simulink model "geuus"  (R2017b)
settings: Solver=VariableStepAuto  StartTime=0.0  StopTime=10.0  RelTol=1e-3
values from neighbouring files (symbols this model uses):
  d2hhh1 = fnval(fnder(fnder(sp1)),vvv1)    [feedbackcontrolcal.m]
  d2hhh2 = fnval(fnder(fnder(sp2)),vvv2)    [feedbackcontrolcal.m]
  dhhh1 = fnval(fnder(sp1),vvv1)    [feedbackcontrolcal.m]
  dhhh2 = fnval(fnder(sp2),vvv2)    [feedbackcontrolcal.m]
  hhh1 = altitude(1:19)*1000    [feedbackcontrolcal.m]
  hhh2 = altitude(19:end)*1000    [feedbackcontrolcal.m]
  vvv1 = speed(1:19)*1000    [feedbackcontrolcal.m]
  vvv2 = speed(19:end)*1000    [feedbackcontrolcal.m]
settings Model: Creator=ztyab  LastModifiedBy=ztyab

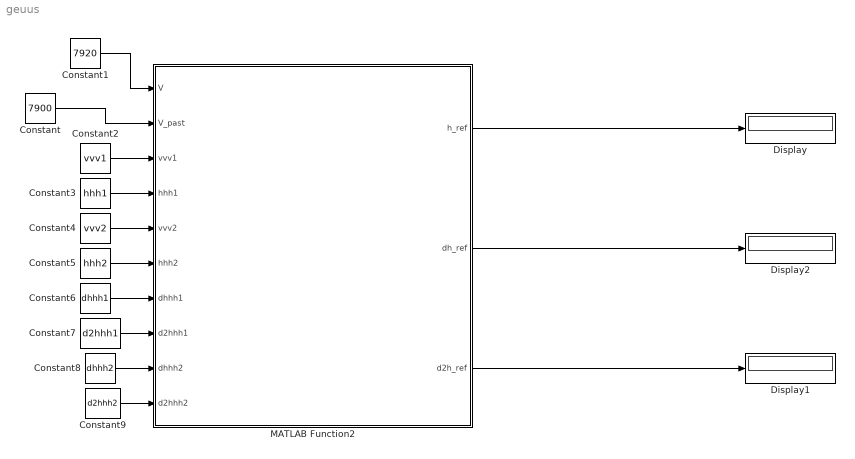
== system geuus ==
  Constant : Constant  Value=7900
  Constant1 : Constant  Value=7920
  Constant2 : Constant  Value=vvv1
  Constant3 : Constant  Value=hhh1
  Constant4 : Constant  Value=vvv2
  Constant5 : Constant  Value=hhh2
  Constant6 : Constant  Value=dhhh1
  Constant7 : Constant  Value=d2hhh1
  Constant8 : Constant  Value=dhhh2
  Constant9 : Constant  Value=d2hhh2
  Display : Display
  Display1 : Display
  Display2 : Display
  MATLAB Function2 : MATLAB Function  TreatAsAtomicUnit=on
  wires:
  Constant/1 -> MATLAB Function2/2(V_past)
  Constant1/1 -> MATLAB Function2/1(V)
  Constant2/1 -> MATLAB Function2/3(vvv1)
  Constant3/1 -> MATLAB Function2/4(hhh1)
  Constant4/1 -> MATLAB Function2/5(vvv2)
  Constant5/1 -> MATLAB Function2/6(hhh2)
  MATLAB Function2/1(h_ref) -> Display/1
  MATLAB Function2/2(dh_ref) -> Display2/1
  MATLAB Function2/3(d2h_ref) -> Display1/1
  Constant6/1 -> MATLAB Function2/7(dhhh1)
  Constant7/1 -> MATLAB Function2/8(d2hhh1)
  Constant8/1 -> MATLAB Function2/9(dhhh2)
  Constant9/1 -> MATLAB Function2/10(d2hhh2)

== matlab function geuus/MATLAB Function2 ==
  data: V input; h_ref output; V_past input; vvv1 input; hhh1 input; vvv2 input; hhh2 input; dh_ref output; d2h_ref output; dhhh1 input; d2hhh1 input; dhhh2 input; d2hhh2 input
function [h_ref,dh_ref,d2h_ref] = fcn(V,V_past,vvv1,hhh1,vvv2,hhh2,dhhh1,d2hhh1,dhhh2,d2hhh2)



if(V>=V_past)
    h_ref1=interp1(vvv1,hhh1,V,'spline');
    dh_ref1=interp1(vvv1,dhhh1,V,'spline');
    d2h_ref1=interp1(vvv1,d2hhh1,V,'spline');
else
    h_ref1=interp1(vvv2,hhh2,V,'spline');
    dh_ref1=interp1(vvv2,dhhh2,V,'spline');
    d2h_ref1=interp1(vvv2,d2hhh2,V,'spline');
end
h_ref=h_ref1;
dh_ref=dh_ref1;
d2h_ref=d2h_ref1;


end
